simulink model "sps_solarcell"  (R2014a)
settings: Solver=ode23tb  StartTime=0.0  StopTime=10  RelTol=1e-3
undefined symbols (not defined in the file or in its folder): Ts
libraries: powerlib x10, simulink x3, simulink_extras x1
settings Model: Creator=cosorio  LastModifiedBy=cosorio
settings DataIOCC: LimitDataPoints=off  SignalLoggingSaveFormat=ModelDataLogs  SaveOutput=off  SignalLogging=off  SaveTime=off
settings OptimizationCC: ExpressionDepthLimit=2147483647
settings DebuggingCC: UnderspecifiedInitializationDetection=Classic  SolverPrmCheckMsg=none  FcnCallInpInsideContextMsg=UseLocalSettings  StateNameClashWarn=warning
settings GRTTargetCC: CombineOutputUpdateFcns=off  GRTInterface=on

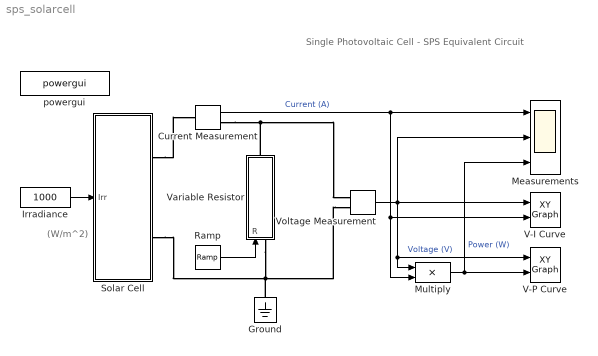
== system sps_solarcell ==
  note: Single Photovoltaic Cell - SPS Equivalent Circuit
  note: (W/m^2)
  Current Measurement : powerlib/Measurements/Current Measurement  PhasorSimulation=off  OutputType=Complex  PSBequivalent=0
  Ground : powerlib/Elements/Ground  LConnTagsString=a
  Irradiance : Constant  Value=1000
  Measurements : Scope  NumInputPorts=3
      settings: YMin=0~0~0  YMax=6~1~3  SaveName=SPSSolarCellData
  Multiply : Product  Inputs=**
  Ramp : simulink/Sources/Ramp  slope=0.1  start=0  X0=0
  Solar Cell : Subsystem
  V-I Curve : simulink/Sinks/XY Graph  xmin=0  xmax=0.6  ymin=0  ymax=6  st=-1
  V-P Curve : simulink/Sinks/XY Graph  xmin=0  xmax=0.6  ymin=0  ymax=3  st=-1
  Variable Resistor : Subsystem  mask(Variable Resistor){tau=1e-4, I0out=5, I0in=0}
      mask prompts: tau "Time constant (sec):"; I0out "Initial Output Current (A):"; I0in "Initial Input Current (A):"
      mask help: This block implements a SimPowerSystems variable resistor using Simulink
  Voltage Measurement : powerlib/Measurements/Voltage Measurement  PhasorSimulation=off  OutputType=Complex  PSBequivalent=0
  powergui : powerlib/powergui  Priority=1  SimulationMode=Continuous  SolverType=Tustin  SampleTime=Ts  frequency=60  SPID=off  DisableSnubberDevices=off  DisableRonSwitches=off  DisableVfSwitches=off  SwTol=0  Interpol=off  DisplayEquations=off  Ts=0  methode=off  frequencyindice=0  Pbase=100e6  ErrMax=1e-4  Iterations=50  UnitsV=kV  UnitsW=MW  FunctionMessages=off  echomessages=off  HookPort=off  EnableUseOfTLC=off  x0status=blocks  RestoreLinks=warning  ResistiveCurrentMeasurement=off  Frange=[0:2:500]  Ylog=off  Xlog=on  ShowGrid=off  save=off  variable=ZData  structure=0  ZoomFFT=on  StartTime=0.0  cycles=1  DisplayStyle=1  fundamental=60  FreqAxis=off  MaxFrequency=1000  frequencyindicesteady=1  RmsSteady=1  display=off
  wires:
  Irradiance/1 -> Solar Cell/1(Irr)
  Current Measurement/1 -> Measurements/1, V-I Curve/2, Multiply/2  "Current (A)"
  Voltage Measurement/1 -> V-I Curve/1, Multiply/1, V-P Curve/1, Measurements/2  "Voltage (V)"
  Multiply/1 -> V-P Curve/2, Measurements/3  "Power (W)"
  Ramp/1 -> Variable Resistor/1(R)
  connections:
  Voltage Measurement/LConn2 -- Variable Resistor/LConn1 -- Ground/LConn1 -- Solar Cell/RConn2
  Current Measurement/RConn1 -- Variable Resistor/RConn1 -- Voltage Measurement/LConn1
  Solar Cell/RConn1 -- Current Measurement/LConn1

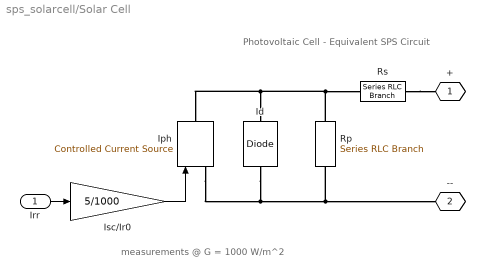
== system sps_solarcell/Solar Cell ==
  note: measurements @ G = 1000 W/m^2
  note: Photovoltaic Cell - Equivalent SPS Circuit
  Irr : Inport
  Id : powerlib/Power Electronics/Diode  Ron=0.02  Lon=0  Vf=0.5  IC=0  UseSnubber=off  Rs=inf  Cs=0  Measurements=off
  Iph : powerlib/Electrical Sources/Controlled Current Source  Initialize=on  Source_Type=AC  Amplitude=0  Phase=0  Frequency=0  Measurements=None
  Isc/Ir0 : Gain  Gain=5/1000
  Rp : powerlib/Elements/Series RLC Branch  LConnTagsString=__new0  RConnTagsString=__new0  BranchType=R  Resistance=1e3  Inductance=1e-3  SetiL0=off  InitialCurrent=0  Capacitance=1e-6  Setx0=off  InitialVoltage=0  Measurements=None
  Rs : powerlib/Elements/Series RLC Branch  LConnTagsString=__new0  RConnTagsString=__new0  BranchType=R  Resistance=.001  Inductance=1e-3  SetiL0=off  InitialCurrent=0  Capacitance=1e-6  Setx0=off  InitialVoltage=0  Measurements=None
  + : PMIOPort  Tag=PMCPort  Port=1  Side=Right
  -- : PMIOPort  Tag=PMCPort  Port=2  Side=Right
  wires:
  Isc/Ir0/1 -> Iph/1
  Irr/1 -> Isc/Ir0/1
  connections:
  Iph/LConn1 -- --/RConn1 -- Rp/RConn1 -- Id/RConn1
  Rp/LConn1 -- Rs/LConn1 -- Iph/RConn1 -- Id/LConn1
  Rs/RConn1 -- +/RConn1

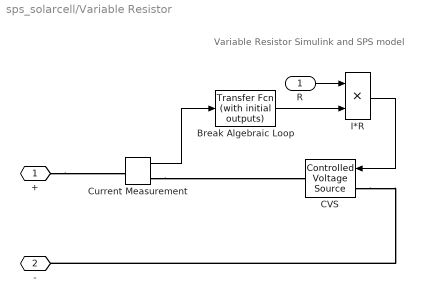
== system sps_solarcell/Variable Resistor ==
  note: Variable Resistor Simulink and SPS model
  R : Inport
  Break Algebraic Loop : simulink_extras/Additional Linear/Transfer Fcn (with initial outputs)  N=[1]  D="[tau  1]"  Y0=I0out  U0=I0in
  CVS : powerlib/Electrical Sources/Controlled Voltage Source  Initialize=on  Source_Type=AC  Amplitude=0  Phase=0  Frequency=0  Measurements=None
  Current Measurement : powerlib/Measurements/Current Measurement  PhasorSimulation=off  OutputType=Complex  PSBequivalent=0
  I*R : Product  Inputs=**
  + : PMIOPort  Port=1  Side=Right
  - : PMIOPort  Port=2  Side=Left
  wires:
  I*R/1 -> CVS/1
  Current Measurement/1 -> Break Algebraic Loop/1
  Break Algebraic Loop/1 -> I*R/2
  R/1 -> I*R/1
  connections:
  Current Measurement/RConn1 -- CVS/RConn1
  +/RConn1 -- Current Measurement/LConn1
  CVS/LConn1 -- -/RConn1
